simulink model "sm_DynamicCompression"  (R2019b)
settings: Solver=FixedStepDiscrete  StartTime=0.0  StopTime=stop_time  RelTol=1e-3
InitFcn:
  | sm_callback_init
StopFcn:
  | sm_callback_stop
values from neighbouring files (symbols this model uses):
  a = 100*(r^2)    [InitializeCompressionSettings.m]    (also in sm_check_control_signals.m = registers(i).(supplied_fields{j}); sm_check_control_signals_LOCAL_1434.m = registers(i).(supplied_fields{j}))
  B_k_0_init = zeros(1,FIR_0_Uprate)    [sm_callback_init.m]
  B_k_1_init = zeros(1,FIR_0_Uprate)    [sm_callback_init.m]
  B_k_2_init = zeros(1,FIR_0_Uprate)    [sm_callback_init.m]
  B_k_3_init = zeros(1,FIR_0_Uprate)    [sm_callback_init.m]
  B_k_4_init = zeros(1,FIR_0_Uprate)    [sm_callback_init.m]
  B_k_5_init = zeros(1,FIR_0_Uprate)    [sm_callback_init.m]
  calib_bpfs = bpfs    [sm_compression_init.m]
  delayFix = maxDelay-delays    [Initialize_Delay_Values.m]
  F_bits = 28    [TestingLibraryScripts.m]    (also in sm_compression_init.m)
  FIR_0_Size = (ceil(log2(length(calib_bpfs(2:calib_bpfs(1,1)+1 ,1)'))))    [sm_callback_init.m]
  FIR_0_Uprate = 2^FIR_0_Size    [sm_callback_init.m]
  M_bits = 1    [TestingLibraryScripts.m]    (also in sm_compression_init.m = 5)
  M_Bits = M_bits    (= 5)    [sm_compression_init.m]
  mp = sm_init_avalon_signals(mp)    [sm_callback_init.m]
  r_att = nthroot(0.1, s_att)    [sm_compression_init.m]
  r_rel = nthroot(0.1, s_rel)    [sm_compression_init.m]
  recombGain = ones(1,NChans)    [sm_compression_init.m]
  TABLE_SEL_BYPASS_ENABLE = 0    [sm_callback_init.m]
  Ts = mp.Ts    [sm_compression_init.m]
  Ts_system = mp.Ts_system    [sm_compression_init.m]
  W_bits = 32    [TestingLibraryScripts.m]    (also in sm_compression_init.m)
  X_high = 1    [sm_compression_init.m]
undefined symbols (not defined in the file or in its folder): b, c, Gain_Table, ig_eq
libraries: hdlsllib x272, simulink x127, dsphdlfiltering x2
(part 4 of 8)

== system sm_DynamicCompression/dataplane/Avalon Data Processing/Left Channel Processing/recalculate/Nchan_FbankAGC_AID/Compression_1/Compression_Gain_Calc/High_Gain_Table ==
  wr_din : Inport
  wr_addr : Inport  Port=2
  wr_en : Inport  Port=3  OutDataTypeStr=boolean
  rd_addr : Inport  Port=4
  Signal Specification : SignalSpecification  OutDataTypeStr=fixdt(0,ram_size,0)  Dimensions=1
  Signal Specification1 : SignalSpecification  OutDataTypeStr=fixdt(0,ram_size,0)  Dimensions=1
  convert : DataTypeConversion  OutDataTypeStr=uint16
  convert1 : DataTypeConversion  OutDataTypeStr=uint16
  ram : UnitDelay  InitialCondition=Gain_Table(:,1)  SampleTime=-1  HasFrameUpgradeWarning=on
  ram_data : UnitDelay  SampleTime=-1  HasFrameUpgradeWarning=on
  select : Selector  IndexMode=Zero-based  InputPortWidth=2^ram_size  IndexOptions=Index vector (port)  Indices=[1 3]  OutputSizes=1
  select1 : Selector  IndexMode=Zero-based  InputPortWidth=2^ram_size  IndexOptions=Index vector (port)  Indices=[1 3]  OutputSizes=1
  switch : Switch  Criteria=u2 ~= 0
  wr_addr_d : UnitDelay  SampleTime=-1  HasFrameUpgradeWarning=on
  wr_port : Assignment  IndexMode=Zero-based  IndexOptions=Index vector (port)  Indices=1  OutputSizes=[1 1]
  wr_dout : Outport  VectorParamsAs1DForOutWhenUnconnected=off
  rd_dout : Outport  Port=2  VectorParamsAs1DForOutWhenUnconnected=off
  wires:
  Signal Specification1/1 -> convert1/1
  wr_addr_d/1 -> select1/2
  select1/1 -> wr_dout/1
  convert1/1 -> select/2
  convert/1 -> wr_addr_d/1, wr_port/3
  select/1 -> ram_data/1
  rd_addr/1 -> Signal Specification1/1
  wr_en/1 -> switch/2
  wr_din/1 -> wr_port/2
  ram/1 -> switch/3, select1/1, select/1, wr_port/1
  switch/1 -> ram/1
  wr_port/1 -> switch/1
  wr_addr/1 -> Signal Specification/1
  Signal Specification/1 -> convert/1
  ram_data/1 -> rd_dout/1

== system sm_DynamicCompression/dataplane/Avalon Data Processing/Left Channel Processing/recalculate/Nchan_FbankAGC_AID/Compression_1/Compression_Gain_Calc/Linear_Approximation ==
  note: Check if |X_in| is less than x_low,
      | if true, use the low gain instead of
      | linear interpolation
  note: NOTE: When NShifts would be > 15, the output gain is slightly too small.
      | This is marginal as this volume is below the threshold, but for consistency,
      | all gains on volumes below the threshold will be set to x_low value, the
      | gain applied to an input of 2^-15
      | Outputs above 85 dBA will be clipped to 85 dBA.
  G_high : Inport
  G_low : Inport  Port=2
  addr_low : Inport  Port=3
  |X_in| : Inport  Port=4
  Bit Rotate1 : hdlsllib/Logic and Bit Operations/Bit Rotate  mode=Rotate Right  N=M_Bits
      settings: SourceProductName=Simulink  SourceProductBaseCode=SL
  Bit Slice : hdlsllib/Logic and Bit Operations/Bit Slice  lidx=M_Bits+3  ridx=M_Bits
      settings: SourceProductName=Simulink  SourceProductBaseCode=SL
  Bit Slice1 : hdlsllib/Logic and Bit Operations/Bit Slice  lidx=M_Bits-1  ridx=0
      settings: SourceProductName=Simulink  SourceProductBaseCode=SL
  Bitwise Operator : simulink/Logic and Bit Operations/Bitwise Operator  logicop=NOT  UseBitMask=off  BitMask=bin2dec('11011001')  BitMaskRealWorld=Stored Integer
  Compare To Constant : simulink/Logic and Bit Operations/Compare To Constant  relop=<  const=0  OutDataTypeStr=boolean
  Constant : Constant  OutDataTypeStr=fixdt(0,W_bits,W_bits-2)  SampleTime=-1
  Constant2 : Constant  Value=2^(M_bits)  OutDataTypeStr=fixdt(0,W_bits,0)  SampleTime=-1
  Data Type Conversion : DataTypeConversion  OutDataTypeStr=fixdt(1,W_bits,F_bits)
  Data Type Conversion1 : DataTypeConversion  OutDataTypeStr=fixdt(1,W_bits, F_bits)
  LSL(N) : Subsystem
  LSR(N) : Subsystem
  Product1 : Product
  Product2 : Product
  Product3 : Product
  Subtract : Sum  Inputs=-+
  Subtract1 : Sum  OutDataTypeStr=fixdt(1,W_bits, F_bits)
  Subtract2 : Sum  Inputs=+-  OutDataTypeStr=Inherit: Same as first input
  Subtract3 : Sum
  Switch : Switch  Criteria=u2 > Threshold
  Unit Delay : UnitDelay  InitialCondition=1  SampleTime=-1  HasFrameUpgradeWarning=on
  G_Desired : Outport  VectorParamsAs1DForOutWhenUnconnected=off
  wires:
  addr_low/1 -> Bit Slice1/1, Bit Slice/1
  Bit Slice/1 -> Bitwise Operator/1
  Bitwise Operator/1 -> LSR(N)/1(NShifts), LSL(N)/1(NShifts)  "NShifts"
  Bit Slice1/1 -> Product1/2  "M"
  G_high/1 -> Subtract/2
  G_low/1 -> Subtract/1, Switch/1, Subtract3/1
  Subtract/1 -> Product2/1  "Delta_G"
  Constant/1 -> LSR(N)/2(x_in)
  LSR(N)/1(x_shifted) -> Bit Rotate1/1, Subtract1/1  "2^(-NShifts)"
  Bit Rotate1/1 -> Product1/1  "2^(-M_bits-NShifts)"
  Product1/1 -> Subtract1/2  "M*2^(-M_bits-NShifts)"
  Subtract1/1 -> Subtract2/2  "x_low"
  LSL(N)/1(x_shifted) -> Product2/2  "1/Delta_x"
  Product2/1 -> Product3/1  "slope"
  |X_in|/1 -> Subtract2/1
  Subtract2/1 -> Compare To Constant/1, Product3/2
  Product3/1 -> Data Type Conversion/1  "M*2^(-2-NShifts)"
  Subtract3/1 -> Data Type Conversion1/1
  Constant2/1 -> LSL(N)/2(x_in)
  Data Type Conversion/1 -> Subtract3/2
  Data Type Conversion1/1 -> Switch/3
  Unit Delay/1 -> G_Desired/1
  Compare To Constant/1 -> Switch/2
  Switch/1 -> Unit Delay/1

== system sm_DynamicCompression/dataplane/Avalon Data Processing/Left Channel Processing/recalculate/Nchan_FbankAGC_AID/Compression_1/Compression_Gain_Calc/LogAddressing ==
  note: Note: simulation version of this block has no latency.
      | But, in VHDL the inputs are registered, delaying the signal by 1.
  note: Have to change size by 8 because LZC made for 40 bit number
  note: EFFECTIVELY shift_left(x_in,NShifts)
  x_in : Inport
  Bit Concat : hdlsllib/Logic and Bit Operations/Bit Concat  numInputs=2
      settings: SourceProductName=Simulink
  Bit Slice : hdlsllib/Logic and Bit Operations/Bit Slice  lidx=3  ridx=0
      settings: SourceProductName=Simulink  SourceProductBaseCode=SL
  Bit Slice1 : hdlsllib/Logic and Bit Operations/Bit Slice  lidx=F_bits-1  ridx=F_bits-M_bits
      settings: SourceProductName=Simulink  SourceProductBaseCode=SL
  Bitwise Operator1 : simulink/Logic and Bit Operations/Bitwise Operator  logicop=NOT  UseBitMask=off  BitMask=bin2dec('11011001')  BitMaskRealWorld=Stored Integer
  Compare To Constant1 : simulink/Logic and Bit Operations/Compare To Constant  relop=>  const=15  OutDataTypeStr=boolean
  Constant1 : Constant  Value=W_bits-1-F_bits  OutDataTypeStr=fixdt(0,6,0)  SampleTime=-1
  Constant6 : Constant  Value=0  OutDataTypeStr=fixdt(0,9,0)  SampleTime=-1
  Data Type Conversion : DataTypeConversion  OutDataTypeStr=fixdt(0,W_bits+8,F_bits+8)
  Data Type Conversion1 : DataTypeConversion  OutDataTypeStr=fixdt(0,W_bits,F_bits)
  Delay2 : Delay  DelayLength=1
  LSL(N) : Subsystem
  MATLAB Function : MATLAB Function  TreatAsAtomicUnit=on
  Subtract : Sum  Inputs=+-  OutDataTypeStr=Inherit: Same as first input
  Switch1 : Switch  Criteria=u2 ~= 0
  fxpt_lzc_W32 : Subsystem  Commented=on  TreatAsAtomicUnit=on
  addr_r : Outport  VectorParamsAs1DForOutWhenUnconnected=off
  wires:
  x_in/1 -> Data Type Conversion/1
  Bit Slice1/1 -> Bit Concat/2  "M"
  Bitwise Operator1/1 -> Bit Concat/1  "addr(5 downto 2)"
  MATLAB Function/1(lzc_count) -> Subtract/1
  Bit Concat/1 -> Switch1/3
  Constant1/1 -> Subtract/2
  Bit Slice/1 -> Bitwise Operator1/1, LSL(N)/1(NShifts)  "NShifts"
  Delay2/1 -> LSL(N)/2(x_in)
  LSL(N)/1(x_shifted) -> Bit Slice1/1
  Data Type Conversion/1 -> MATLAB Function/1(x), Data Type Conversion1/1
  Constant6/1 -> Switch1/1
  Switch1/1 -> addr_r/1
  Compare To Constant1/1 -> Switch1/2
  Subtract/1 -> Compare To Constant1/1, Bit Slice/1
  Data Type Conversion1/1 -> Delay2/1

== system sm_DynamicCompression/dataplane/Avalon Data Processing/Left Channel Processing/recalculate/Nchan_FbankAGC_AID/Compression_1/Compression_Gain_Calc/Low_Gain_Table ==
  note: Initialized
  wr_din : Inport
  wr_addr : Inport  Port=2
  wr_en : Inport  Port=3  OutDataTypeStr=boolean
  rd_addr : Inport  Port=4
  Signal Specification : SignalSpecification  OutDataTypeStr=fixdt(0,ram_size,0)  Dimensions=1
  Signal Specification1 : SignalSpecification  OutDataTypeStr=fixdt(0,ram_size,0)  Dimensions=1
  convert : DataTypeConversion  OutDataTypeStr=uint16
  convert1 : DataTypeConversion  OutDataTypeStr=uint16
  ram : UnitDelay  InitialCondition=Gain_Table(:,1)  SampleTime=-1  HasFrameUpgradeWarning=on
  ram_data : UnitDelay  SampleTime=-1  HasFrameUpgradeWarning=on
  select : Selector  IndexMode=Zero-based  InputPortWidth=2^ram_size  IndexOptions=Index vector (port)  Indices=[1 3]  OutputSizes=1
  select1 : Selector  IndexMode=Zero-based  InputPortWidth=2^ram_size  IndexOptions=Index vector (port)  Indices=[1 3]  OutputSizes=1
  switch : Switch  Criteria=u2 ~= 0
  wr_addr_d : UnitDelay  SampleTime=-1  HasFrameUpgradeWarning=on
  wr_port : Assignment  IndexMode=Zero-based  IndexOptions=Index vector (port)  Indices=1  OutputSizes=[1 1]
  wr_dout : Outport  VectorParamsAs1DForOutWhenUnconnected=off
  rd_dout : Outport  Port=2  VectorParamsAs1DForOutWhenUnconnected=off
  wires:
  ram_data/1 -> rd_dout/1
  Signal Specification/1 -> convert/1
  wr_addr/1 -> Signal Specification/1
  wr_port/1 -> switch/1
  switch/1 -> ram/1
  ram/1 -> wr_port/1, select/1, select1/1, switch/3
  wr_din/1 -> wr_port/2
  wr_en/1 -> switch/2
  rd_addr/1 -> Signal Specification1/1
  select/1 -> ram_data/1
  convert/1 -> wr_port/3, wr_addr_d/1
  convert1/1 -> select/2
  select1/1 -> wr_dout/1
  wr_addr_d/1 -> select1/2
  Signal Specification1/1 -> convert1/1

== system sm_DynamicCompression/dataplane/Avalon Data Processing/Left Channel Processing/recalculate/Nchan_FbankAGC_AID/Compression_2/Compression_Envelope/Attack_Envelope ==
  note: ATTACK
  Curr : Inport
  Desired : Inport  Port=2
  Enable : EnablePort
  Product : Product  OutDataTypeStr=Inherit: Same as first input
  Subtract : Sum  Inputs=+-
  Subtract1 : Sum  OutDataTypeStr=fixdt(1,W_bits, F_bits)
  r_att(2) : Constant  Value=r_att(2)  OutDataTypeStr=fixdt(1,W_bits*2,W_bits+F_bits)  SampleTime=-1
  Gain_out : Outport  InitialOutput=0  VectorParamsAs1DForOutWhenUnconnected=off
  wires:
  Desired/1 -> Subtract/2, Subtract1/2
  Curr/1 -> Subtract/1
  Subtract/1 -> Product/2
  r_att(2)/1 -> Product/1
  Product/1 -> Subtract1/1  "Apply_Envelope"
  Subtract1/1 -> Gain_out/1

== system sm_DynamicCompression/dataplane/Avalon Data Processing/Left Channel Processing/recalculate/Nchan_FbankAGC_AID/Compression_2/Compression_Envelope/Release_Envelope ==
  note: RELEASE
  Curr : Inport
  Desired : Inport  Port=2
  Enable : EnablePort
  Product : Product  OutDataTypeStr=Inherit: Same as first input
  Subtract : Sum  Inputs=+-
  Subtract1 : Sum  Inputs=+-  OutDataTypeStr=Inherit: Same as first input
  r_rel(2) : Constant  Value=r_rel(2)  OutDataTypeStr=fixdt(1,W_bits*2,W_bits+F_bits)  SampleTime=-1
  Gain_out : Outport  InitialOutput=0  VectorParamsAs1DForOutWhenUnconnected=off
  wires:
  Desired/1 -> Subtract1/1, Subtract/1
  Curr/1 -> Subtract/2
  Subtract/1 -> Product/1
  r_rel(2)/1 -> Product/2
  Product/1 -> Subtract1/2  "Apply_Envelope"
  Subtract1/1 -> Gain_out/1

== system sm_DynamicCompression/dataplane/Avalon Data Processing/Left Channel Processing/recalculate/Nchan_FbankAGC_AID/Compression_2/Compression_Gain_Calc/High_Gain_Table ==
  wr_din : Inport
  wr_addr : Inport  Port=2
  wr_en : Inport  Port=3  OutDataTypeStr=boolean
  rd_addr : Inport  Port=4
  Signal Specification : SignalSpecification  OutDataTypeStr=fixdt(0,ram_size,0)  Dimensions=1
  Signal Specification1 : SignalSpecification  OutDataTypeStr=fixdt(0,ram_size,0)  Dimensions=1
  convert : DataTypeConversion  OutDataTypeStr=uint16
  convert1 : DataTypeConversion  OutDataTypeStr=uint16
  ram : UnitDelay  InitialCondition=Gain_Table(:,2)  SampleTime=-1  HasFrameUpgradeWarning=on
  ram_data : UnitDelay  SampleTime=-1  HasFrameUpgradeWarning=on
  select : Selector  IndexMode=Zero-based  InputPortWidth=2^ram_size  IndexOptions=Index vector (port)  Indices=[1 3]  OutputSizes=1
  select1 : Selector  IndexMode=Zero-based  InputPortWidth=2^ram_size  IndexOptions=Index vector (port)  Indices=[1 3]  OutputSizes=1
  switch : Switch  Criteria=u2 ~= 0
  wr_addr_d : UnitDelay  SampleTime=-1  HasFrameUpgradeWarning=on
  wr_port : Assignment  IndexMode=Zero-based  IndexOptions=Index vector (port)  Indices=1  OutputSizes=[1 1]
  wr_dout : Outport  VectorParamsAs1DForOutWhenUnconnected=off
  rd_dout : Outport  Port=2  VectorParamsAs1DForOutWhenUnconnected=off
  wires:
  Signal Specification1/1 -> convert1/1
  wr_addr_d/1 -> select1/2
  select1/1 -> wr_dout/1
  convert1/1 -> select/2
  convert/1 -> wr_addr_d/1, wr_port/3
  select/1 -> ram_data/1
  rd_addr/1 -> Signal Specification1/1
  wr_en/1 -> switch/2
  wr_din/1 -> wr_port/2
  ram/1 -> switch/3, select1/1, select/1, wr_port/1
  switch/1 -> ram/1
  wr_port/1 -> switch/1
  wr_addr/1 -> Signal Specification/1
  Signal Specification/1 -> convert/1
  ram_data/1 -> rd_dout/1

== system sm_DynamicCompression/dataplane/Avalon Data Processing/Left Channel Processing/recalculate/Nchan_FbankAGC_AID/Compression_2/Compression_Gain_Calc/Linear_Approximation ==
  note: Check if |X_in| is less than x_low,
      | if true, use the low gain instead of
      | linear interpolation
  note: NOTE: When NShifts would be > 15, the output gain is slightly too small.
      | This is marginal as this volume is below the threshold, but for consistency,
      | all gains on volumes below the threshold will be set to x_low value, the
      | gain applied to an input of 2^-15
      | Outputs above 85 dBA will be clipped to 85 dBA.
  G_high : Inport
  G_low : Inport  Port=2
  addr_low : Inport  Port=3
  |X_in| : Inport  Port=4
  Bit Rotate1 : hdlsllib/Logic and Bit Operations/Bit Rotate  mode=Rotate Right  N=M_Bits
      settings: SourceProductName=Simulink  SourceProductBaseCode=SL
  Bit Slice : hdlsllib/Logic and Bit Operations/Bit Slice  lidx=M_Bits+3  ridx=M_Bits
      settings: SourceProductName=Simulink  SourceProductBaseCode=SL
  Bit Slice1 : hdlsllib/Logic and Bit Operations/Bit Slice  lidx=M_Bits-1  ridx=0
      settings: SourceProductName=Simulink  SourceProductBaseCode=SL
  Bitwise Operator : simulink/Logic and Bit Operations/Bitwise Operator  logicop=NOT  UseBitMask=off  BitMask=bin2dec('11011001')  BitMaskRealWorld=Stored Integer
  Compare To Constant : simulink/Logic and Bit Operations/Compare To Constant  relop=<  const=0  OutDataTypeStr=boolean
  Constant : Constant  OutDataTypeStr=fixdt(0,W_bits,W_bits-2)  SampleTime=-1
  Constant2 : Constant  Value=2^(M_bits)  OutDataTypeStr=fixdt(0,W_bits,0)  SampleTime=-1
  Data Type Conversion : DataTypeConversion  OutDataTypeStr=fixdt(1,W_bits,F_bits)
  Data Type Conversion1 : DataTypeConversion  OutDataTypeStr=fixdt(1,W_bits, F_bits)
  LSL(N) : Subsystem
  LSR(N) : Subsystem
  Product1 : Product
  Product2 : Product
  Product3 : Product
  Subtract : Sum  Inputs=-+
  Subtract1 : Sum  OutDataTypeStr=fixdt(1,W_bits, F_bits)
  Subtract2 : Sum  Inputs=+-  OutDataTypeStr=Inherit: Same as first input
  Subtract3 : Sum
  Switch : Switch  Criteria=u2 > Threshold
  Unit Delay : UnitDelay  InitialCondition=1  SampleTime=-1  HasFrameUpgradeWarning=on
  G_Desired : Outport  VectorParamsAs1DForOutWhenUnconnected=off
  wires:
  addr_low/1 -> Bit Slice1/1, Bit Slice/1
  Bit Slice/1 -> Bitwise Operator/1
  Bitwise Operator/1 -> LSR(N)/1(NShifts), LSL(N)/1(NShifts)  "NShifts"
  Bit Slice1/1 -> Product1/2  "M"
  G_high/1 -> Subtract/2
  G_low/1 -> Subtract/1, Switch/1, Subtract3/1
  Subtract/1 -> Product2/1  "Delta_G"
  Constant/1 -> LSR(N)/2(x_in)
  LSR(N)/1(x_shifted) -> Bit Rotate1/1, Subtract1/1  "2^(-NShifts)"
  Bit Rotate1/1 -> Product1/1  "2^(-M_bits-NShifts)"
  Product1/1 -> Subtract1/2  "M*2^(-M_bits-NShifts)"
  Subtract1/1 -> Subtract2/2  "x_low"
  LSL(N)/1(x_shifted) -> Product2/2  "1/Delta_x"
  Product2/1 -> Product3/1  "slope"
  |X_in|/1 -> Subtract2/1
  Subtract2/1 -> Compare To Constant/1, Product3/2
  Product3/1 -> Data Type Conversion/1  "M*2^(-2-NShifts)"
  Subtract3/1 -> Data Type Conversion1/1
  Constant2/1 -> LSL(N)/2(x_in)
  Data Type Conversion/1 -> Subtract3/2
  Data Type Conversion1/1 -> Switch/3
  Unit Delay/1 -> G_Desired/1
  Compare To Constant/1 -> Switch/2
  Switch/1 -> Unit Delay/1

== system sm_DynamicCompression/dataplane/Avalon Data Processing/Left Channel Processing/recalculate/Nchan_FbankAGC_AID/Compression_2/Compression_Gain_Calc/LogAddressing ==
  note: Note: simulation version of this block has no latency.
      | But, in VHDL the inputs are registered, delaying the signal by 1.
  note: Have to change size by 8 because LZC made for 40 bit number
  note: EFFECTIVELY shift_left(x_in,NShifts)
  x_in : Inport
  Bit Concat : hdlsllib/Logic and Bit Operations/Bit Concat  numInputs=2
      settings: SourceProductName=Simulink
  Bit Slice : hdlsllib/Logic and Bit Operations/Bit Slice  lidx=3  ridx=0
      settings: SourceProductName=Simulink  SourceProductBaseCode=SL
  Bit Slice1 : hdlsllib/Logic and Bit Operations/Bit Slice  lidx=F_bits-1  ridx=F_bits-M_bits
      settings: SourceProductName=Simulink  SourceProductBaseCode=SL
  Bitwise Operator1 : simulink/Logic and Bit Operations/Bitwise Operator  logicop=NOT  UseBitMask=off  BitMask=bin2dec('11011001')  BitMaskRealWorld=Stored Integer
  Compare To Constant1 : simulink/Logic and Bit Operations/Compare To Constant  relop=>  const=15  OutDataTypeStr=boolean
  Constant1 : Constant  Value=W_bits-1-F_bits  OutDataTypeStr=fixdt(0,6,0)  SampleTime=-1
  Constant6 : Constant  Value=0  OutDataTypeStr=fixdt(0,9,0)  SampleTime=-1
  Data Type Conversion : DataTypeConversion  OutDataTypeStr=fixdt(0,W_bits+8,F_bits+8)
  Data Type Conversion1 : DataTypeConversion  OutDataTypeStr=fixdt(0,W_bits,F_bits)
  Delay2 : Delay  DelayLength=1
  LSL(N) : Subsystem
  MATLAB Function : MATLAB Function  TreatAsAtomicUnit=on
  Subtract : Sum  Inputs=+-  OutDataTypeStr=Inherit: Same as first input
  Switch1 : Switch  Criteria=u2 ~= 0
  addr_r : Outport  VectorParamsAs1DForOutWhenUnconnected=off
  wires:
  x_in/1 -> Data Type Conversion/1
  Bit Slice1/1 -> Bit Concat/2  "M"
  Bitwise Operator1/1 -> Bit Concat/1  "addr(5 downto 2)"
  MATLAB Function/1(lzc_count) -> Subtract/1
  Bit Concat/1 -> Switch1/3
  Constant1/1 -> Subtract/2
  Bit Slice/1 -> Bitwise Operator1/1, LSL(N)/1(NShifts)  "NShifts"
  Delay2/1 -> LSL(N)/2(x_in)
  LSL(N)/1(x_shifted) -> Bit Slice1/1
  Data Type Conversion/1 -> MATLAB Function/1(x), Data Type Conversion1/1
  Constant6/1 -> Switch1/1
  Switch1/1 -> addr_r/1
  Compare To Constant1/1 -> Switch1/2
  Subtract/1 -> Compare To Constant1/1, Bit Slice/1
  Data Type Conversion1/1 -> Delay2/1

== system sm_DynamicCompression/dataplane/Avalon Data Processing/Left Channel Processing/recalculate/Nchan_FbankAGC_AID/Compression_2/Compression_Gain_Calc/Low_Gain_Table ==
  wr_din : Inport
  wr_addr : Inport  Port=2
  wr_en : Inport  Port=3  OutDataTypeStr=boolean
  rd_addr : Inport  Port=4
  Signal Specification : SignalSpecification  OutDataTypeStr=fixdt(0,ram_size,0)  Dimensions=1
  Signal Specification1 : SignalSpecification  OutDataTypeStr=fixdt(0,ram_size,0)  Dimensions=1
  convert : DataTypeConversion  OutDataTypeStr=uint16
  convert1 : DataTypeConversion  OutDataTypeStr=uint16
  ram : UnitDelay  InitialCondition=Gain_Table(:,2)  SampleTime=-1  HasFrameUpgradeWarning=on
  ram_data : UnitDelay  SampleTime=-1  HasFrameUpgradeWarning=on
  select : Selector  IndexMode=Zero-based  InputPortWidth=2^ram_size  IndexOptions=Index vector (port)  Indices=[1 3]  OutputSizes=1
  select1 : Selector  IndexMode=Zero-based  InputPortWidth=2^ram_size  IndexOptions=Index vector (port)  Indices=[1 3]  OutputSizes=1
  switch : Switch  Criteria=u2 ~= 0
  wr_addr_d : UnitDelay  SampleTime=-1  HasFrameUpgradeWarning=on
  wr_port : Assignment  IndexMode=Zero-based  IndexOptions=Index vector (port)  Indices=1  OutputSizes=[1 1]
  wr_dout : Outport  VectorParamsAs1DForOutWhenUnconnected=off
  rd_dout : Outport  Port=2  VectorParamsAs1DForOutWhenUnconnected=off
  wires:
  ram_data/1 -> rd_dout/1
  Signal Specification/1 -> convert/1
  wr_addr/1 -> Signal Specification/1
  wr_port/1 -> switch/1
  switch/1 -> ram/1
  ram/1 -> wr_port/1, select/1, select1/1, switch/3
  wr_din/1 -> wr_port/2
  wr_en/1 -> switch/2
  rd_addr/1 -> Signal Specification1/1
  select/1 -> ram_data/1
  convert/1 -> wr_port/3, wr_addr_d/1
  convert1/1 -> select/2
  select1/1 -> wr_dout/1
  wr_addr_d/1 -> select1/2
  Signal Specification1/1 -> convert1/1

== system sm_DynamicCompression/dataplane/Avalon Data Processing/Left Channel Processing/recalculate/Nchan_FbankAGC_AID/Compression_3/Compression_Envelope/Attack_Envelope ==
  note: ATTACK
  Curr : Inport
  Desired : Inport  Port=2
  Enable : EnablePort
  Product : Product  OutDataTypeStr=Inherit: Same as first input
  Subtract : Sum  Inputs=+-
  Subtract1 : Sum  OutDataTypeStr=fixdt(1,W_bits, F_bits)
  r_att(3) : Constant  Value=r_att(3)  OutDataTypeStr=fixdt(1,W_bits*2,W_bits+F_bits)  SampleTime=-1
  Gain_out : Outport  InitialOutput=0  VectorParamsAs1DForOutWhenUnconnected=off
  wires:
  Desired/1 -> Subtract/2, Subtract1/2
  Curr/1 -> Subtract/1
  Subtract/1 -> Product/2
  r_att(3)/1 -> Product/1
  Product/1 -> Subtract1/1  "Apply_Envelope"
  Subtract1/1 -> Gain_out/1

== system sm_DynamicCompression/dataplane/Avalon Data Processing/Left Channel Processing/recalculate/Nchan_FbankAGC_AID/Compression_3/Compression_Envelope/Release_Envelope ==
  note: RELEASE
  Curr : Inport
  Desired : Inport  Port=2
  Enable : EnablePort
  Product : Product  OutDataTypeStr=Inherit: Same as first input
  Subtract : Sum  Inputs=+-
  Subtract1 : Sum  Inputs=+-  OutDataTypeStr=Inherit: Same as first input
  r_rel(3) : Constant  Value=r_rel(3)  OutDataTypeStr=fixdt(1,W_bits*2,W_bits+F_bits)  SampleTime=-1
  Gain_out : Outport  InitialOutput=0  VectorParamsAs1DForOutWhenUnconnected=off
  wires:
  Desired/1 -> Subtract1/1, Subtract/1
  Curr/1 -> Subtract/2
  Subtract/1 -> Product/1
  r_rel(3)/1 -> Product/2
  Product/1 -> Subtract1/2  "Apply_Envelope"
  Subtract1/1 -> Gain_out/1

== system sm_DynamicCompression/dataplane/Avalon Data Processing/Left Channel Processing/recalculate/Nchan_FbankAGC_AID/Compression_3/Compression_Gain_Calc/High_Gain_Table ==
  wr_din : Inport
  wr_addr : Inport  Port=2
  wr_en : Inport  Port=3  OutDataTypeStr=boolean
  rd_addr : Inport  Port=4
  Signal Specification : SignalSpecification  OutDataTypeStr=fixdt(0,ram_size,0)  Dimensions=1
  Signal Specification1 : SignalSpecification  OutDataTypeStr=fixdt(0,ram_size,0)  Dimensions=1
  convert : DataTypeConversion  OutDataTypeStr=uint16
  convert1 : DataTypeConversion  OutDataTypeStr=uint16
  ram : UnitDelay  InitialCondition=Gain_Table(:,3)  SampleTime=-1  HasFrameUpgradeWarning=on
  ram_data : UnitDelay  SampleTime=-1  HasFrameUpgradeWarning=on
  select : Selector  IndexMode=Zero-based  InputPortWidth=2^ram_size  IndexOptions=Index vector (port)  Indices=[1 3]  OutputSizes=1
  select1 : Selector  IndexMode=Zero-based  InputPortWidth=2^ram_size  IndexOptions=Index vector (port)  Indices=[1 3]  OutputSizes=1
  switch : Switch  Criteria=u2 ~= 0
  wr_addr_d : UnitDelay  SampleTime=-1  HasFrameUpgradeWarning=on
  wr_port : Assignment  IndexMode=Zero-based  IndexOptions=Index vector (port)  Indices=1  OutputSizes=[1 1]
  wr_dout : Outport  VectorParamsAs1DForOutWhenUnconnected=off
  rd_dout : Outport  Port=2  VectorParamsAs1DForOutWhenUnconnected=off
  wires:
  Signal Specification1/1 -> convert1/1
  wr_addr_d/1 -> select1/2
  select1/1 -> wr_dout/1
  convert1/1 -> select/2
  convert/1 -> wr_addr_d/1, wr_port/3
  select/1 -> ram_data/1
  rd_addr/1 -> Signal Specification1/1
  wr_en/1 -> switch/2
  wr_din/1 -> wr_port/2
  ram/1 -> switch/3, select1/1, select/1, wr_port/1
  switch/1 -> ram/1
  wr_port/1 -> switch/1
  wr_addr/1 -> Signal Specification/1
  Signal Specification/1 -> convert/1
  ram_data/1 -> rd_dout/1

== system sm_DynamicCompression/dataplane/Avalon Data Processing/Left Channel Processing/recalculate/Nchan_FbankAGC_AID/Compression_3/Compression_Gain_Calc/Linear_Approximation ==
  note: Check if |X_in| is less than x_low,
      | if true, use the low gain instead of
      | linear interpolation
  note: NOTE: When NShifts would be > 15, the output gain is slightly too small.
      | This is marginal as this volume is below the threshold, but for consistency,
      | all gains on volumes below the threshold will be set to x_low value, the
      | gain applied to an input of 2^-15
      | Outputs above 85 dBA will be clipped to 85 dBA.
  G_high : Inport
  G_low : Inport  Port=2
  addr_low : Inport  Port=3
  |X_in| : Inport  Port=4
  Bit Rotate1 : hdlsllib/Logic and Bit Operations/Bit Rotate  mode=Rotate Right  N=M_Bits
      settings: SourceProductName=Simulink  SourceProductBaseCode=SL
  Bit Slice : hdlsllib/Logic and Bit Operations/Bit Slice  lidx=M_Bits+3  ridx=M_Bits
      settings: SourceProductName=Simulink  SourceProductBaseCode=SL
  Bit Slice1 : hdlsllib/Logic and Bit Operations/Bit Slice  lidx=M_Bits-1  ridx=0
      settings: SourceProductName=Simulink  SourceProductBaseCode=SL
  Bitwise Operator : simulink/Logic and Bit Operations/Bitwise Operator  logicop=NOT  UseBitMask=off  BitMask=bin2dec('11011001')  BitMaskRealWorld=Stored Integer
  Compare To Constant : simulink/Logic and Bit Operations/Compare To Constant  relop=<  const=0  OutDataTypeStr=boolean
  Constant : Constant  OutDataTypeStr=fixdt(0,W_bits,W_bits-2)  SampleTime=-1
  Constant2 : Constant  Value=2^(M_bits)  OutDataTypeStr=fixdt(0,W_bits,0)  SampleTime=-1
  Data Type Conversion : DataTypeConversion  OutDataTypeStr=fixdt(1,W_bits,F_bits)
  Data Type Conversion1 : DataTypeConversion  OutDataTypeStr=fixdt(1,W_bits, F_bits)
  LSL(N) : Subsystem
  LSR(N) : Subsystem
  Product1 : Product
  Product2 : Product
  Product3 : Product
  Subtract : Sum  Inputs=-+
  Subtract1 : Sum  OutDataTypeStr=fixdt(1,W_bits, F_bits)
  Subtract2 : Sum  Inputs=+-  OutDataTypeStr=Inherit: Same as first input
  Subtract3 : Sum
  Switch : Switch  Criteria=u2 > Threshold
  Unit Delay : UnitDelay  InitialCondition=1  SampleTime=-1  HasFrameUpgradeWarning=on
  G_Desired : Outport  VectorParamsAs1DForOutWhenUnconnected=off
  wires:
  addr_low/1 -> Bit Slice1/1, Bit Slice/1
  Bit Slice/1 -> Bitwise Operator/1
  Bitwise Operator/1 -> LSR(N)/1(NShifts), LSL(N)/1(NShifts)  "NShifts"
  Bit Slice1/1 -> Product1/2  "M"
  G_high/1 -> Subtract/2
  G_low/1 -> Subtract/1, Switch/1, Subtract3/1
  Subtract/1 -> Product2/1  "Delta_G"
  Constant/1 -> LSR(N)/2(x_in)
  LSR(N)/1(x_shifted) -> Bit Rotate1/1, Subtract1/1  "2^(-NShifts)"
  Bit Rotate1/1 -> Product1/1  "2^(-M_bits-NShifts)"
  Product1/1 -> Subtract1/2  "M*2^(-M_bits-NShifts)"
  Subtract1/1 -> Subtract2/2  "x_low"
  LSL(N)/1(x_shifted) -> Product2/2  "1/Delta_x"
  Product2/1 -> Product3/1  "slope"
  |X_in|/1 -> Subtract2/1
  Subtract2/1 -> Compare To Constant/1, Product3/2
  Product3/1 -> Data Type Conversion/1  "M*2^(-2-NShifts)"
  Subtract3/1 -> Data Type Conversion1/1
  Constant2/1 -> LSL(N)/2(x_in)
  Data Type Conversion/1 -> Subtract3/2
  Data Type Conversion1/1 -> Switch/3
  Unit Delay/1 -> G_Desired/1
  Compare To Constant/1 -> Switch/2
  Switch/1 -> Unit Delay/1

== system sm_DynamicCompression/dataplane/Avalon Data Processing/Left Channel Processing/recalculate/Nchan_FbankAGC_AID/Compression_3/Compression_Gain_Calc/LogAddressing ==
  note: Note: simulation version of this block has no latency.
      | But, in VHDL the inputs are registered, delaying the signal by 1.
  note: Have to change size by 8 because LZC made for 40 bit number
  note: EFFECTIVELY shift_left(x_in,NShifts)
  x_in : Inport
  Bit Concat : hdlsllib/Logic and Bit Operations/Bit Concat  numInputs=2
      settings: SourceProductName=Simulink
  Bit Slice : hdlsllib/Logic and Bit Operations/Bit Slice  lidx=3  ridx=0
      settings: SourceProductName=Simulink  SourceProductBaseCode=SL
  Bit Slice1 : hdlsllib/Logic and Bit Operations/Bit Slice  lidx=F_bits-1  ridx=F_bits-M_bits
      settings: SourceProductName=Simulink  SourceProductBaseCode=SL
  Bitwise Operator1 : simulink/Logic and Bit Operations/Bitwise Operator  logicop=NOT  UseBitMask=off  BitMask=bin2dec('11011001')  BitMaskRealWorld=Stored Integer
  Compare To Constant1 : simulink/Logic and Bit Operations/Compare To Constant  relop=>  const=15  OutDataTypeStr=boolean
  Constant1 : Constant  Value=W_bits-1-F_bits  OutDataTypeStr=fixdt(0,6,0)  SampleTime=-1
  Constant6 : Constant  Value=0  OutDataTypeStr=fixdt(0,9,0)  SampleTime=-1
  Data Type Conversion : DataTypeConversion  OutDataTypeStr=fixdt(0,W_bits+8,F_bits+8)
  Data Type Conversion1 : DataTypeConversion  OutDataTypeStr=fixdt(0,W_bits,F_bits)
  Delay2 : Delay  DelayLength=1
  LSL(N) : Subsystem
  MATLAB Function : MATLAB Function  TreatAsAtomicUnit=on
  Subtract : Sum  Inputs=+-  OutDataTypeStr=Inherit: Same as first input
  Switch1 : Switch  Criteria=u2 ~= 0
  addr_r : Outport  VectorParamsAs1DForOutWhenUnconnected=off
  wires:
  x_in/1 -> Data Type Conversion/1
  Bit Slice1/1 -> Bit Concat/2  "M"
  Bitwise Operator1/1 -> Bit Concat/1  "addr(5 downto 2)"
  MATLAB Function/1(lzc_count) -> Subtract/1
  Bit Concat/1 -> Switch1/3
  Constant1/1 -> Subtract/2
  Bit Slice/1 -> Bitwise Operator1/1, LSL(N)/1(NShifts)  "NShifts"
  Delay2/1 -> LSL(N)/2(x_in)
  LSL(N)/1(x_shifted) -> Bit Slice1/1
  Data Type Conversion/1 -> MATLAB Function/1(x), Data Type Conversion1/1
  Constant6/1 -> Switch1/1
  Switch1/1 -> addr_r/1
  Compare To Constant1/1 -> Switch1/2
  Subtract/1 -> Compare To Constant1/1, Bit Slice/1
  Data Type Conversion1/1 -> Delay2/1

== system sm_DynamicCompression/dataplane/Avalon Data Processing/Left Channel Processing/recalculate/Nchan_FbankAGC_AID/Compression_3/Compression_Gain_Calc/Low_Gain_Table ==
  wr_din : Inport
  wr_addr : Inport  Port=2
  wr_en : Inport  Port=3  OutDataTypeStr=boolean
  rd_addr : Inport  Port=4
  Signal Specification : SignalSpecification  OutDataTypeStr=fixdt(0,ram_size,0)  Dimensions=1
  Signal Specification1 : SignalSpecification  OutDataTypeStr=fixdt(0,ram_size,0)  Dimensions=1
  convert : DataTypeConversion  OutDataTypeStr=uint16
  convert1 : DataTypeConversion  OutDataTypeStr=uint16
  ram : UnitDelay  InitialCondition=Gain_Table(:,3)  SampleTime=-1  HasFrameUpgradeWarning=on
  ram_data : UnitDelay  SampleTime=-1  HasFrameUpgradeWarning=on
  select : Selector  IndexMode=Zero-based  InputPortWidth=2^ram_size  IndexOptions=Index vector (port)  Indices=[1 3]  OutputSizes=1
  select1 : Selector  IndexMode=Zero-based  InputPortWidth=2^ram_size  IndexOptions=Index vector (port)  Indices=[1 3]  OutputSizes=1
  switch : Switch  Criteria=u2 ~= 0
  wr_addr_d : UnitDelay  SampleTime=-1  HasFrameUpgradeWarning=on
  wr_port : Assignment  IndexMode=Zero-based  IndexOptions=Index vector (port)  Indices=1  OutputSizes=[1 1]
  wr_dout : Outport  VectorParamsAs1DForOutWhenUnconnected=off
  rd_dout : Outport  Port=2  VectorParamsAs1DForOutWhenUnconnected=off
  wires:
  ram_data/1 -> rd_dout/1
  Signal Specification/1 -> convert/1
  wr_addr/1 -> Signal Specification/1
  wr_port/1 -> switch/1
  switch/1 -> ram/1
  ram/1 -> wr_port/1, select/1, select1/1, switch/3
  wr_din/1 -> wr_port/2
  wr_en/1 -> switch/2
  rd_addr/1 -> Signal Specification1/1
  select/1 -> ram_data/1
  convert/1 -> wr_port/3, wr_addr_d/1
  convert1/1 -> select/2
  select1/1 -> wr_dout/1
  wr_addr_d/1 -> select1/2
  Signal Specification1/1 -> convert1/1

== system sm_DynamicCompression/dataplane/Avalon Data Processing/Left Channel Processing/recalculate/Nchan_FbankAGC_AID/Compression_4/Compression_Envelope/Attack_Envelope ==
  note: ATTACK
  Curr : Inport
  Desired : Inport  Port=2
  Enable : EnablePort
  Product : Product  OutDataTypeStr=Inherit: Same as first input
  Subtract : Sum  Inputs=+-
  Subtract1 : Sum  OutDataTypeStr=fixdt(1,W_bits, F_bits)
  r_att(4) : Constant  Value=r_att(4)  OutDataTypeStr=fixdt(1,W_bits*2,W_bits+F_bits)  SampleTime=-1
  Gain_out : Outport  InitialOutput=0  VectorParamsAs1DForOutWhenUnconnected=off
  wires:
  Desired/1 -> Subtract/2, Subtract1/2
  Curr/1 -> Subtract/1
  Subtract/1 -> Product/2
  r_att(4)/1 -> Product/1
  Product/1 -> Subtract1/1  "Apply_Envelope"
  Subtract1/1 -> Gain_out/1

== system sm_DynamicCompression/dataplane/Avalon Data Processing/Left Channel Processing/recalculate/Nchan_FbankAGC_AID/Compression_4/Compression_Envelope/Release_Envelope ==
  note: RELEASE
  Curr : Inport
  Desired : Inport  Port=2
  Enable : EnablePort
  Product : Product  OutDataTypeStr=Inherit: Same as first input
  Subtract : Sum  Inputs=+-
  Subtract1 : Sum  Inputs=+-  OutDataTypeStr=Inherit: Same as first input
  r_rel(4) : Constant  Value=r_rel(4)  OutDataTypeStr=fixdt(1,W_bits*2,W_bits+F_bits)  SampleTime=-1
  Gain_out : Outport  InitialOutput=0  VectorParamsAs1DForOutWhenUnconnected=off
  wires:
  Desired/1 -> Subtract1/1, Subtract/1
  Curr/1 -> Subtract/2
  Subtract/1 -> Product/1
  r_rel(4)/1 -> Product/2
  Product/1 -> Subtract1/2  "Apply_Envelope"
  Subtract1/1 -> Gain_out/1

== system sm_DynamicCompression/dataplane/Avalon Data Processing/Left Channel Processing/recalculate/Nchan_FbankAGC_AID/Compression_4/Compression_Gain_Calc/High_Gain_Table ==
  wr_din : Inport
  wr_addr : Inport  Port=2
  wr_en : Inport  Port=3  OutDataTypeStr=boolean
  rd_addr : Inport  Port=4
  Signal Specification : SignalSpecification  OutDataTypeStr=fixdt(0,ram_size,0)  Dimensions=1
  Signal Specification1 : SignalSpecification  OutDataTypeStr=fixdt(0,ram_size,0)  Dimensions=1
  convert : DataTypeConversion  OutDataTypeStr=uint16
  convert1 : DataTypeConversion  OutDataTypeStr=uint16
  ram : UnitDelay  InitialCondition=Gain_Table(:,4)  SampleTime=-1  HasFrameUpgradeWarning=on
  ram_data : UnitDelay  SampleTime=-1  HasFrameUpgradeWarning=on
  select : Selector  IndexMode=Zero-based  InputPortWidth=2^ram_size  IndexOptions=Index vector (port)  Indices=[1 3]  OutputSizes=1
  select1 : Selector  IndexMode=Zero-based  InputPortWidth=2^ram_size  IndexOptions=Index vector (port)  Indices=[1 3]  OutputSizes=1
  switch : Switch  Criteria=u2 ~= 0
  wr_addr_d : UnitDelay  SampleTime=-1  HasFrameUpgradeWarning=on
  wr_port : Assignment  IndexMode=Zero-based  IndexOptions=Index vector (port)  Indices=1  OutputSizes=[1 1]
  wr_dout : Outport  VectorParamsAs1DForOutWhenUnconnected=off
  rd_dout : Outport  Port=2  VectorParamsAs1DForOutWhenUnconnected=off
  wires:
  Signal Specification1/1 -> convert1/1
  wr_addr_d/1 -> select1/2
  select1/1 -> wr_dout/1
  convert1/1 -> select/2
  convert/1 -> wr_addr_d/1, wr_port/3
  select/1 -> ram_data/1
  rd_addr/1 -> Signal Specification1/1
  wr_en/1 -> switch/2
  wr_din/1 -> wr_port/2
  ram/1 -> switch/3, select1/1, select/1, wr_port/1
  switch/1 -> ram/1
  wr_port/1 -> switch/1
  wr_addr/1 -> Signal Specification/1
  Signal Specification/1 -> convert/1
  ram_data/1 -> rd_dout/1

== system sm_DynamicCompression/dataplane/Avalon Data Processing/Left Channel Processing/recalculate/Nchan_FbankAGC_AID/Compression_4/Compression_Gain_Calc/Linear_Approximation ==
  note: Check if |X_in| is less than x_low,
      | if true, use the low gain instead of
      | linear interpolation
  note: NOTE: When NShifts would be > 15, the output gain is slightly too small.
      | This is marginal as this volume is below the threshold, but for consistency,
      | all gains on volumes below the threshold will be set to x_low value, the
      | gain applied to an input of 2^-15
      | Outputs above 85 dBA will be clipped to 85 dBA.
  G_high : Inport
  G_low : Inport  Port=2
  addr_low : Inport  Port=3
  |X_in| : Inport  Port=4
  Bit Rotate1 : hdlsllib/Logic and Bit Operations/Bit Rotate  mode=Rotate Right  N=M_Bits
      settings: SourceProductName=Simulink  SourceProductBaseCode=SL
  Bit Slice : hdlsllib/Logic and Bit Operations/Bit Slice  lidx=M_Bits+3  ridx=M_Bits
      settings: SourceProductName=Simulink  SourceProductBaseCode=SL
  Bit Slice1 : hdlsllib/Logic and Bit Operations/Bit Slice  lidx=M_Bits-1  ridx=0
      settings: SourceProductName=Simulink  SourceProductBaseCode=SL
  Bitwise Operator : simulink/Logic and Bit Operations/Bitwise Operator  logicop=NOT  UseBitMask=off  BitMask=bin2dec('11011001')  BitMaskRealWorld=Stored Integer
  Compare To Constant : simulink/Logic and Bit Operations/Compare To Constant  relop=<  const=0  OutDataTypeStr=boolean
  Constant : Constant  OutDataTypeStr=fixdt(0,W_bits,W_bits-2)  SampleTime=-1
  Constant2 : Constant  Value=2^(M_bits)  OutDataTypeStr=fixdt(0,W_bits,0)  SampleTime=-1
  Data Type Conversion : DataTypeConversion  OutDataTypeStr=fixdt(1,W_bits,F_bits)
  Data Type Conversion1 : DataTypeConversion  OutDataTypeStr=fixdt(1,W_bits, F_bits)
  LSL(N) : Subsystem
  LSR(N) : Subsystem
  Product1 : Product
  Product2 : Product
  Product3 : Product
  Subtract : Sum  Inputs=-+
  Subtract1 : Sum  OutDataTypeStr=fixdt(1,W_bits, F_bits)
  Subtract2 : Sum  Inputs=+-  OutDataTypeStr=Inherit: Same as first input
  Subtract3 : Sum
  Switch : Switch  Criteria=u2 > Threshold
  Unit Delay : UnitDelay  InitialCondition=1  SampleTime=-1  HasFrameUpgradeWarning=on
  G_Desired : Outport  VectorParamsAs1DForOutWhenUnconnected=off
  wires:
  addr_low/1 -> Bit Slice1/1, Bit Slice/1
  Bit Slice/1 -> Bitwise Operator/1
  Bitwise Operator/1 -> LSR(N)/1(NShifts), LSL(N)/1(NShifts)  "NShifts"
  Bit Slice1/1 -> Product1/2  "M"
  G_high/1 -> Subtract/2
  G_low/1 -> Subtract/1, Switch/1, Subtract3/1
  Subtract/1 -> Product2/1  "Delta_G"
  Constant/1 -> LSR(N)/2(x_in)
  LSR(N)/1(x_shifted) -> Bit Rotate1/1, Subtract1/1  "2^(-NShifts)"
  Bit Rotate1/1 -> Product1/1  "2^(-M_bits-NShifts)"
  Product1/1 -> Subtract1/2  "M*2^(-M_bits-NShifts)"
  Subtract1/1 -> Subtract2/2  "x_low"
  LSL(N)/1(x_shifted) -> Product2/2  "1/Delta_x"
  Product2/1 -> Product3/1  "slope"
  |X_in|/1 -> Subtract2/1
  Subtract2/1 -> Compare To Constant/1, Product3/2
  Product3/1 -> Data Type Conversion/1  "M*2^(-2-NShifts)"
  Subtract3/1 -> Data Type Conversion1/1
  Constant2/1 -> LSL(N)/2(x_in)
  Data Type Conversion/1 -> Subtract3/2
  Data Type Conversion1/1 -> Switch/3
  Unit Delay/1 -> G_Desired/1
  Compare To Constant/1 -> Switch/2
  Switch/1 -> Unit Delay/1

== system sm_DynamicCompression/dataplane/Avalon Data Processing/Left Channel Processing/recalculate/Nchan_FbankAGC_AID/Compression_4/Compression_Gain_Calc/LogAddressing ==
  note: Note: simulation version of this block has no latency.
      | But, in VHDL the inputs are registered, delaying the signal by 1.
  note: Have to change size by 8 because LZC made for 40 bit number
  note: EFFECTIVELY shift_left(x_in,NShifts)
  x_in : Inport
  Bit Concat : hdlsllib/Logic and Bit Operations/Bit Concat  numInputs=2
      settings: SourceProductName=Simulink
  Bit Slice : hdlsllib/Logic and Bit Operations/Bit Slice  lidx=3  ridx=0
      settings: SourceProductName=Simulink  SourceProductBaseCode=SL
  Bit Slice1 : hdlsllib/Logic and Bit Operations/Bit Slice  lidx=F_bits-1  ridx=F_bits-M_bits
      settings: SourceProductName=Simulink  SourceProductBaseCode=SL
  Bitwise Operator1 : simulink/Logic and Bit Operations/Bitwise Operator  logicop=NOT  UseBitMask=off  BitMask=bin2dec('11011001')  BitMaskRealWorld=Stored Integer
  Compare To Constant1 : simulink/Logic and Bit Operations/Compare To Constant  relop=>  const=15  OutDataTypeStr=boolean
  Constant1 : Constant  Value=W_bits-1-F_bits  OutDataTypeStr=fixdt(0,6,0)  SampleTime=-1
  Constant6 : Constant  Value=0  OutDataTypeStr=fixdt(0,9,0)  SampleTime=-1
  Data Type Conversion : DataTypeConversion  OutDataTypeStr=fixdt(0,W_bits+8,F_bits+8)
  Data Type Conversion1 : DataTypeConversion  OutDataTypeStr=fixdt(0,W_bits,F_bits)
  Delay2 : Delay  DelayLength=1
  LSL(N) : Subsystem
  MATLAB Function : MATLAB Function  TreatAsAtomicUnit=on
  Subtract : Sum  Inputs=+-  OutDataTypeStr=Inherit: Same as first input
  Switch1 : Switch  Criteria=u2 ~= 0
  addr_r : Outport  VectorParamsAs1DForOutWhenUnconnected=off
  wires:
  x_in/1 -> Data Type Conversion/1
  Bit Slice1/1 -> Bit Concat/2  "M"
  Bitwise Operator1/1 -> Bit Concat/1  "addr(5 downto 2)"
  MATLAB Function/1(lzc_count) -> Subtract/1
  Bit Concat/1 -> Switch1/3
  Constant1/1 -> Subtract/2
  Bit Slice/1 -> Bitwise Operator1/1, LSL(N)/1(NShifts)  "NShifts"
  Delay2/1 -> LSL(N)/2(x_in)
  LSL(N)/1(x_shifted) -> Bit Slice1/1
  Data Type Conversion/1 -> MATLAB Function/1(x), Data Type Conversion1/1
  Constant6/1 -> Switch1/1
  Switch1/1 -> addr_r/1
  Compare To Constant1/1 -> Switch1/2
  Subtract/1 -> Compare To Constant1/1, Bit Slice/1
  Data Type Conversion1/1 -> Delay2/1

== system sm_DynamicCompression/dataplane/Avalon Data Processing/Left Channel Processing/recalculate/Nchan_FbankAGC_AID/Compression_4/Compression_Gain_Calc/Low_Gain_Table ==
  wr_din : Inport
  wr_addr : Inport  Port=2
  wr_en : Inport  Port=3  OutDataTypeStr=boolean
  rd_addr : Inport  Port=4
  Signal Specification : SignalSpecification  OutDataTypeStr=fixdt(0,ram_size,0)  Dimensions=1
  Signal Specification1 : SignalSpecification  OutDataTypeStr=fixdt(0,ram_size,0)  Dimensions=1
  convert : DataTypeConversion  OutDataTypeStr=uint16
  convert1 : DataTypeConversion  OutDataTypeStr=uint16
  ram : UnitDelay  InitialCondition=Gain_Table(:,4)  SampleTime=-1  HasFrameUpgradeWarning=on
  ram_data : UnitDelay  SampleTime=-1  HasFrameUpgradeWarning=on
  select : Selector  IndexMode=Zero-based  InputPortWidth=2^ram_size  IndexOptions=Index vector (port)  Indices=[1 3]  OutputSizes=1
  select1 : Selector  IndexMode=Zero-based  InputPortWidth=2^ram_size  IndexOptions=Index vector (port)  Indices=[1 3]  OutputSizes=1
  switch : Switch  Criteria=u2 ~= 0
  wr_addr_d : UnitDelay  SampleTime=-1  HasFrameUpgradeWarning=on
  wr_port : Assignment  IndexMode=Zero-based  IndexOptions=Index vector (port)  Indices=1  OutputSizes=[1 1]
  wr_dout : Outport  VectorParamsAs1DForOutWhenUnconnected=off
  rd_dout : Outport  Port=2  VectorParamsAs1DForOutWhenUnconnected=off
  wires:
  ram_data/1 -> rd_dout/1
  Signal Specification/1 -> convert/1
  wr_addr/1 -> Signal Specification/1
  wr_port/1 -> switch/1
  switch/1 -> ram/1
  ram/1 -> wr_port/1, select/1, select1/1, switch/3
  wr_din/1 -> wr_port/2
  wr_en/1 -> switch/2
  rd_addr/1 -> Signal Specification1/1
  select/1 -> ram_data/1
  convert/1 -> wr_port/3, wr_addr_d/1
  convert1/1 -> select/2
  select1/1 -> wr_dout/1
  wr_addr_d/1 -> select1/2
  Signal Specification1/1 -> convert1/1

== system sm_DynamicCompression/dataplane/Avalon Data Processing/Left Channel Processing/recalculate/Nchan_FbankAGC_AID/Compression_5/Compression_Envelope/Attack_Envelope ==
  note: ATTACK
  Curr : Inport
  Desired : Inport  Port=2
  Enable : EnablePort
  Product : Product  OutDataTypeStr=Inherit: Same as first input
  Subtract : Sum  Inputs=+-
  Subtract1 : Sum  OutDataTypeStr=fixdt(1,W_bits, F_bits)
  r_att(5) : Constant  Value=r_att(5)  OutDataTypeStr=fixdt(1,W_bits*2,W_bits+F_bits)  SampleTime=-1
  Gain_out : Outport  InitialOutput=0  VectorParamsAs1DForOutWhenUnconnected=off
  wires:
  Desired/1 -> Subtract/2, Subtract1/2
  Curr/1 -> Subtract/1
  Subtract/1 -> Product/2
  r_att(5)/1 -> Product/1
  Product/1 -> Subtract1/1  "Apply_Envelope"
  Subtract1/1 -> Gain_out/1

== system sm_DynamicCompression/dataplane/Avalon Data Processing/Left Channel Processing/recalculate/Nchan_FbankAGC_AID/Compression_5/Compression_Envelope/Release_Envelope ==
  note: RELEASE
  Curr : Inport
  Desired : Inport  Port=2
  Enable : EnablePort
  Product : Product  OutDataTypeStr=Inherit: Same as first input
  Subtract : Sum  Inputs=+-
  Subtract1 : Sum  Inputs=+-  OutDataTypeStr=Inherit: Same as first input
  r_rel(5) : Constant  Value=r_rel(5)  OutDataTypeStr=fixdt(1,W_bits*2,W_bits+F_bits)  SampleTime=-1
  Gain_out : Outport  InitialOutput=0  VectorParamsAs1DForOutWhenUnconnected=off
  wires:
  Desired/1 -> Subtract1/1, Subtract/1
  Curr/1 -> Subtract/2
  Subtract/1 -> Product/1
  r_rel(5)/1 -> Product/2
  Product/1 -> Subtract1/2  "Apply_Envelope"
  Subtract1/1 -> Gain_out/1

== system sm_DynamicCompression/dataplane/Avalon Data Processing/Left Channel Processing/recalculate/Nchan_FbankAGC_AID/Compression_5/Compression_Gain_Calc/High_Gain_Table ==
  wr_din : Inport
  wr_addr : Inport  Port=2
  wr_en : Inport  Port=3  OutDataTypeStr=boolean
  rd_addr : Inport  Port=4
  Signal Specification : SignalSpecification  OutDataTypeStr=fixdt(0,ram_size,0)  Dimensions=1
  Signal Specification1 : SignalSpecification  OutDataTypeStr=fixdt(0,ram_size,0)  Dimensions=1
  convert : DataTypeConversion  OutDataTypeStr=uint16
  convert1 : DataTypeConversion  OutDataTypeStr=uint16
  ram : UnitDelay  InitialCondition=Gain_Table(:,5)  SampleTime=-1  HasFrameUpgradeWarning=on
  ram_data : UnitDelay  SampleTime=-1  HasFrameUpgradeWarning=on
  select : Selector  IndexMode=Zero-based  InputPortWidth=2^ram_size  IndexOptions=Index vector (port)  Indices=[1 3]  OutputSizes=1
  select1 : Selector  IndexMode=Zero-based  InputPortWidth=2^ram_size  IndexOptions=Index vector (port)  Indices=[1 3]  OutputSizes=1
  switch : Switch  Criteria=u2 ~= 0
  wr_addr_d : UnitDelay  SampleTime=-1  HasFrameUpgradeWarning=on
  wr_port : Assignment  IndexMode=Zero-based  IndexOptions=Index vector (port)  Indices=1  OutputSizes=[1 1]
  wr_dout : Outport  VectorParamsAs1DForOutWhenUnconnected=off
  rd_dout : Outport  Port=2  VectorParamsAs1DForOutWhenUnconnected=off
  wires:
  Signal Specification1/1 -> convert1/1
  wr_addr_d/1 -> select1/2
  select1/1 -> wr_dout/1
  convert1/1 -> select/2
  convert/1 -> wr_addr_d/1, wr_port/3
  select/1 -> ram_data/1
  rd_addr/1 -> Signal Specification1/1
  wr_en/1 -> switch/2
  wr_din/1 -> wr_port/2
  ram/1 -> switch/3, select1/1, select/1, wr_port/1
  switch/1 -> ram/1
  wr_port/1 -> switch/1
  wr_addr/1 -> Signal Specification/1
  Signal Specification/1 -> convert/1
  ram_data/1 -> rd_dout/1
